simulink model "cv_3"  (R2022a)
settings: Solver=VariableStepAuto  StartTime=0.0  StopTime=10  MaxStep=1e-3  RelTol=1e-3
values from neighbouring files (symbols this model uses):
  b = 0.1    [cv_3.m]
  F_a = 1    [cv_3.m]
  k = 500    [cv_3.m]
  m = 2    [cv_3.m]
  w = 2*pi*10    (= 62.8318530718)    [cv_3.m]
undefined symbols (not defined in the file or in its folder): I, M_h, M_z
libraries: simulink x2
settings Model: Creator=221208  LastModifiedBy=221208

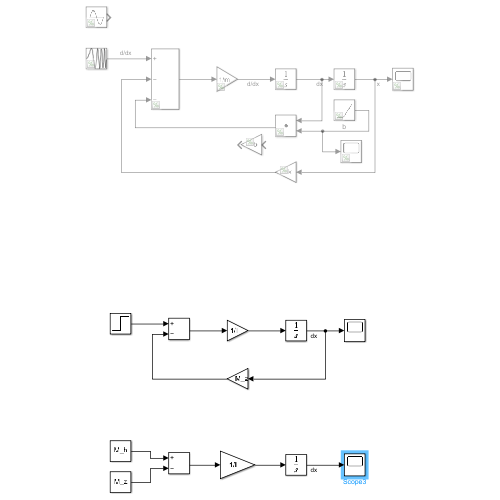
[thumbnail: Simulink's stored preview of the top-level diagram]
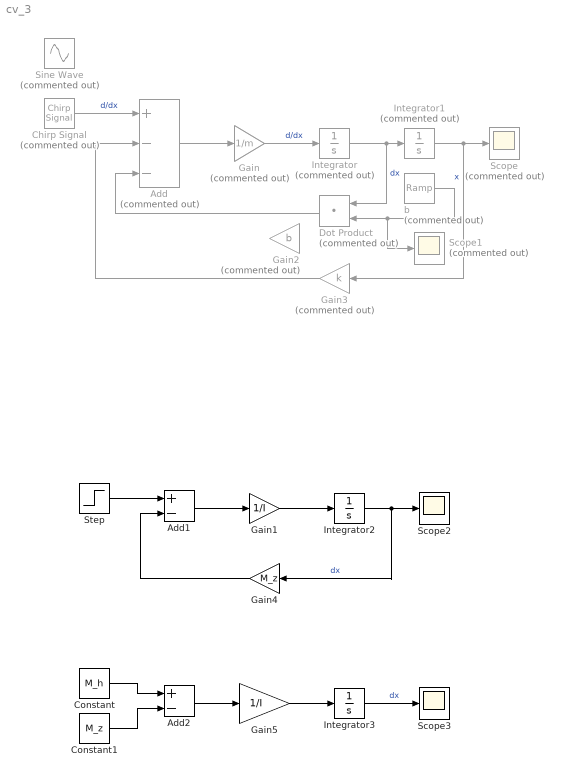
== system cv_3 ==
  Add : Sum  Commented=on  Inputs=+--
  Add1 : Sum  Inputs=+-
  Add2 : Sum  Inputs=+-
  Chirp Signal : simulink/Sources/Chirp Signal  Commented=on  f1=0  T=100  f2=100
  Constant : Constant  Value=M_h
  Constant1 : Constant  Value=M_z
  Dot Product : DotProduct  Commented=on  OutDataTypeStr=Inherit: Inherit via internal rule
  Gain : Gain  Commented=on  Gain=1/m
  Gain1 : Gain  Gain=1/I
  Gain2 : Gain  Commented=on  Gain=b
  Gain3 : Gain  Commented=on  Gain=k
  Gain4 : Gain  Gain=M_z
  Gain5 : Gain  Gain=1/I
  Integrator : Integrator  Commented=on
  Integrator1 : Integrator  Commented=on
  Integrator2 : Integrator
  Integrator3 : Integrator
  Scope : Scope  Commented=on
  Scope1 : Scope  Commented=on
  Scope2 : Scope
  Scope3 : Scope
  Sine Wave : Sin  Commented=on  Amplitude=F_a  Frequency=w  SampleTime=0
  Step : Step  After=M_h  SampleTime=0
  b : simulink/Sources/Ramp  Commented=on  slope=1  start=40  InitialOutput=0.1
  wires:
  Gain/1 -> Integrator/1  "d/dx"
  Integrator/1 -> Integrator1/1, Dot Product/1  "dx"
  Integrator1/1 -> Gain3/1, Scope/1  "x"
  Chirp Signal/1 -> Add/1  "d/dx"
  Add/1 -> Gain/1
  Gain3/1 -> Add/2
  b/1 -> Scope1/1, Dot Product/2
  Dot Product/1 -> Add/3
  Gain1/1 -> Integrator2/1
  Integrator2/1 -> Gain4/1, Scope2/1  "dx"
  Step/1 -> Add1/1
  Add1/1 -> Gain1/1
  Gain4/1 -> Add1/2
  Integrator3/1 -> Scope3/1  "dx"
  Gain5/1 -> Integrator3/1
  Add2/1 -> Gain5/1
  Constant1/1 -> Add2/2
  Constant/1 -> Add2/1
